simulink model "JKFFStateDiagram"  (R2025b)
settings: Solver=VariableStepAuto  StartTime=0.0  StopTime=inf  RelTol=1e-3
libraries: simulink_extras x1
settings Model: PacingRate=11  Creator=Soochan Kim  LastModifiedBy=Soochan Kim

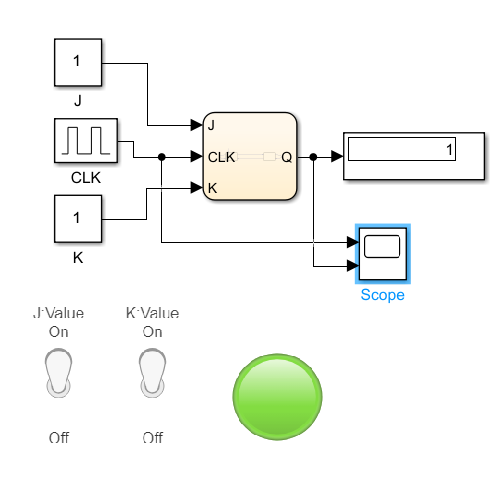
[thumbnail: Simulink's stored preview of the top-level diagram]
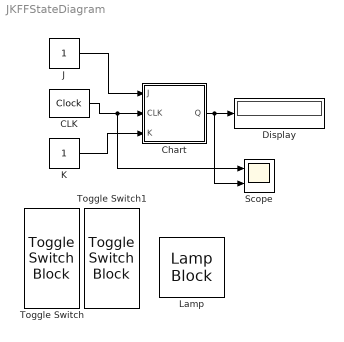
== system JKFFStateDiagram ==
  CLK : simulink_extras/Flip Flops/Clock  period=0.5
  Chart : Stateflow chart  TreatAsAtomicUnit=on
  Display : Display
  J : Constant
  K : Constant
  Lamp : LampBlock  LabelPosition=Hide  DefaultColor=[192.0, 192.0, 192.0]
  Scope : Scope  NumInputPorts=2
      settings: ActiveDisplayYMinimum=-0.125  ActiveDisplayYMaximum=1.125
  Toggle Switch : ToggleSwitchBlock
  Toggle Switch1 : ToggleSwitchBlock
  wires:
  J/1 -> Chart/1(J)
  K/1 -> Chart/3(K)
  CLK/1 -> Scope/1, Chart/2(CLK)
  Chart/1(Q) -> Scope/2, Display/1

== stateflow chart JKFFStateDiagram/Chart ==
  state State_Q0
    entry:
    Q=0;
    notQ=1;
  state State_Q1
    entry:
    Q=1;
    notQ=0;
  (default) -> State_Q0
  State_Q0 -> State_Q1 [order 1] : [rising(CLK) && J==1]
  State_Q1 -> State_Q1 [order 2] : [rising(CLK) && K==0]
  State_Q0 -> State_Q0 [order 2] : [rising(CLK) && J==0]
  State_Q1 -> State_Q0 [order 1] : [rising(CLK) && K==1]
  data: J input; Q output; notQ local; CLK input; K input
